simulink model "ljsduffing"  (Simulink 4.00)
settings: Solver=ode45  SolverMode=SingleTasking  StartTime=34  StopTime=300  RelTol=1e-3  AbsTol=1e-6
libraries: simulink3 x1
settings Model: LastModifiedBy=LJS  LimitDataPoints=off

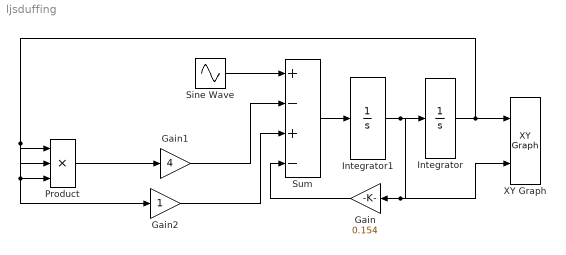
== system ljsduffing ==
  Gain : Gain  Orientation=left  Gain=0.154  Multiplication=Element-wise(K.*u)  SaturateOnIntegerOverflow=on
  Gain1 : Gain  Gain=4  Multiplication=Element-wise(K.*u)  SaturateOnIntegerOverflow=on
  Gain2 : Gain  Gain=1  Multiplication=Element-wise(K.*u)  SaturateOnIntegerOverflow=on
  Integrator : Integrator  ExternalReset=none  InitialConditionSource=internal  InitialCondition=1  LimitOutput=off  UpperSaturationLimit=inf  LowerSaturationLimit=-inf  ShowSaturationPort=off  ShowStatePort=off  AbsoluteTolerance=auto
  Integrator1 : Integrator  ExternalReset=none  InitialConditionSource=internal  InitialCondition=1  LimitOutput=off  UpperSaturationLimit=inf  LowerSaturationLimit=-inf  ShowSaturationPort=off  ShowStatePort=off  AbsoluteTolerance=auto
  Product : Product  Inputs=3  Multiplication=Element-wise(.*)  SaturateOnIntegerOverflow=on
  Sine Wave : Sin  SineType=Time-based  Amplitude=0.150825  Bias=0  Frequency=1.1  Phase=0  Samples=10  SampleTime=0  Offset=0
  Sum : Sum  Inputs=+-+-  SaturateOnIntegerOverflow=on
  XY Graph : simulink3/Sinks/XY Graph  xmin=-1.5  xmax=1.5  ymin=-1.5  ymax=1.5  st=0.01
  wires:
  Sine Wave/1 -> Sum/1
  Sum/1 -> Integrator1/1
  Product/1 -> Gain1/1
  Gain1/1 -> Sum/2
  Gain2/1 -> Sum/3
  Gain/1 -> Sum/4
  Integrator1/1 -> Integrator/1, Gain/1, XY Graph/2
  Integrator/1 -> XY Graph/1, Product/1, Product/2, Product/3, Gain2/1
